simulink model "lab7_t29"  (R2021a)
settings: Solver=VariableStepAuto  StartTime=0.0  StopTime=10.0  RelTol=1e-3
libraries: simulink x1
settings Model: Creator=reemb  LastModifiedBy=reemb

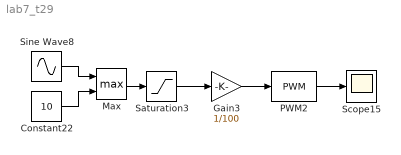
== system lab7_t29 ==
  Constant22 : Constant  Value=10
  Gain3 : Gain  Gain=1/100
  Max : MinMax  Function=max  Inputs=2
  PWM2 : simulink/Discontinuities/PWM  DisableCoverage=on  Period=1  DisallowZeroDutyCycle=off  RunAtFixedTimeIntervals=off  SampleTime=0.1
  Saturation3 : Saturate  UpperLimit=90  LowerLimit=0
  Scope15 : Scope
  Sine Wave8 : Sin  SampleTime=0
  wires:
  PWM2/1 -> Scope15/1
  Saturation3/1 -> Gain3/1
  Sine Wave8/1 -> Max/1
  Gain3/1 -> PWM2/1
  Max/1 -> Saturation3/1
  Constant22/1 -> Max/2
